simulink model "HConstfolding_export_orig"  (Simulink 7.9)
settings: Solver=ode3  StartTime=0.0  StopTime=100000000.0  FixedStep=1  RelTol=1e-3
settings Model: Creator=boakes  LastModifiedBy=boakes

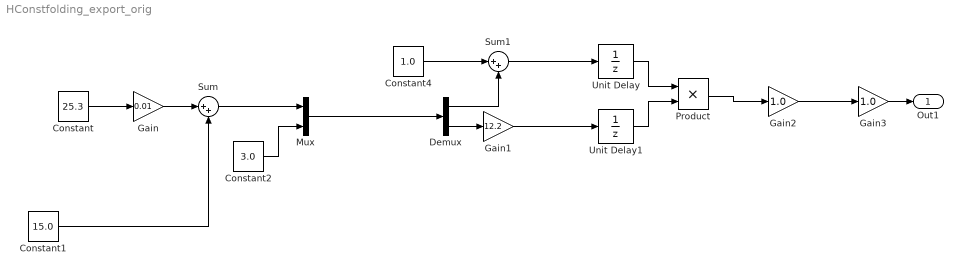
== system HConstfolding_export_orig ==
  Constant : Constant  Value=25.3
  Constant1 : Constant  Value=15.0
  Constant2 : Constant  Value=3.0
  Constant4 : Constant  Value=1.0
  Demux : Demux  Outputs=2
  Gain : Gain  Gain=0.01
  Gain1 : Gain  Gain=12.2
  Gain2 : Gain  Gain=1.0
  Gain3 : Gain  Gain=1.0
  Mux : Mux  Inputs=2
  Product : Product  RndMeth=Zero
  Sum : Sum  Inputs=|++
  Sum1 : Sum  Inputs=|++
  Unit Delay : UnitDelay  X0=0.0  SampleTime=-1.0
  Unit Delay1 : UnitDelay  X0=0.0  SampleTime=-1.0
  Out1 : Outport
  wires:
  Gain2/1 -> Gain3/1
  Product/1 -> Gain2/1
  Constant/1 -> Gain/1
  Gain3/1 -> Out1/1
  Gain1/1 -> Unit Delay1/1
  Sum/1 -> Mux/1
  Unit Delay1/1 -> Product/2
  Mux/1 -> Demux/1
  Sum1/1 -> Unit Delay/1
  Unit Delay/1 -> Product/1
  Gain/1 -> Sum/1
  Demux/1 -> Sum1/2
  Demux/2 -> Gain1/1
  Constant4/1 -> Sum1/1
  Constant1/1 -> Sum/2
  Constant2/1 -> Mux/2
